simulink model "uvms_kinematics"  (Simulink 7.9)
settings: Solver=ode3  StartTime=0.0  StopTime=10.0  FixedStep=dt  RelTol=1e-3
values from neighbouring files (symbols this model uses):
  DH = struct('a',zeros(n,1),'d',zeros(n,1),'alpha',zeros(n,1))    [init.m]
  dt = 0.01    [run_simulation.m]
  VV_States = struct('StatusLinear',0, 'StatusAngular', 0 ,'Circle2EEVec',zeros(3,1), 'linearVehicleVelocity', zeros(6,1),                     'angularVehicleVelocity', zeros(6,1) , 'psibe',0, 'V_EE', zeros(6,1), 'VdotP',0)    [run_simulation.m]
undefined symbols (not defined in the file or in its folder): CircleProps, ee_pose_init, ee_pose_quaternion_init, q_init, QLimits, vehicle_euler_init, vehicle_position_init
libraries: simulink x6
settings Model: Creator=simena  LastModifiedBy=simena
settings DebuggingCC: UnderspecifiedInitializationDetection=Simplified

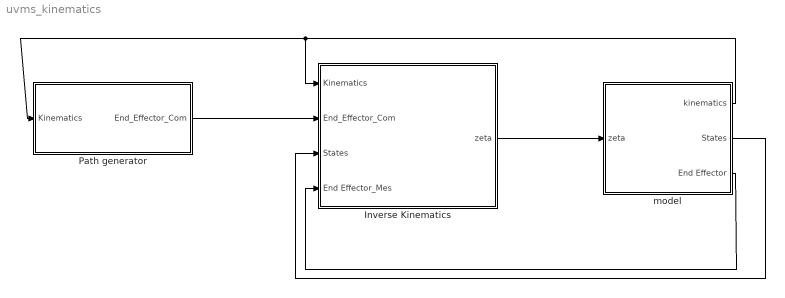
== system uvms_kinematics ==
  Inverse Kinematics : Subsystem
  Path generator : Subsystem
  model : Subsystem
  wires:
  Inverse Kinematics/1(zeta) -> model/1(zeta)
  model/1(kinematics) -> Inverse Kinematics/1(Kinematics), Path generator/1(Kinematics)
  model/3(End Effector) -> Inverse Kinematics/4(End Effector_Mes)
  Path generator/1(End_Effector_Com) -> Inverse Kinematics/2(End_Effector_Com)
  model/2(States) -> Inverse Kinematics/3(States)

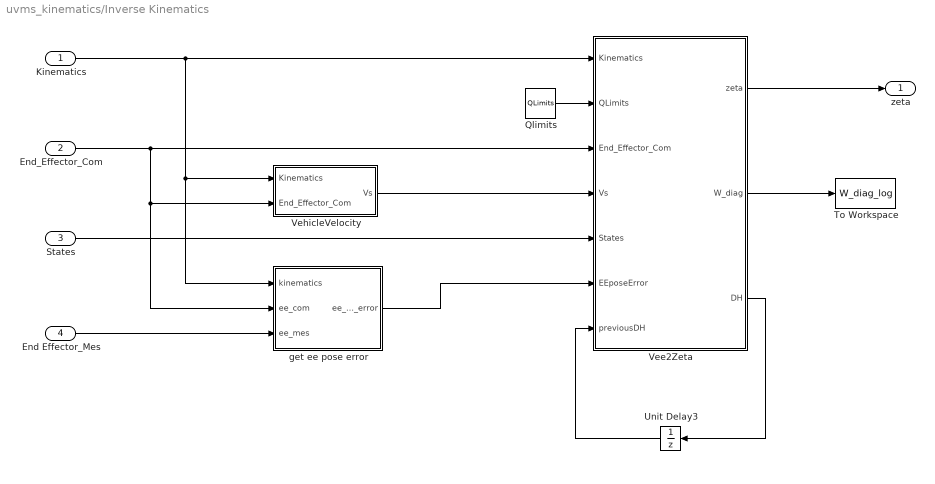
== system uvms_kinematics/Inverse Kinematics ==
  Kinematics : Inport
  End_Effector_Com : Inport  Port=2
  States : Inport  Port=3
  End Effector_Mes : Inport  Port=4
  Qlimits : Constant  Value=QLimits  OutDataTypeStr=Bus: qlimits_bus
  To Workspace : ToWorkspace  VariableName=W_diag_log  SampleTime=-1  SaveFormat=Timeseries
  Unit Delay3 : UnitDelay  X0=zeros(12,12)  SampleTime=-1
  Vee2Zeta : MATLAB Function  TreatAsAtomicUnit=on  SystemSampleTime=dt
  VehicleVelocity : Subsystem
  get ee pose error : Subsystem
  zeta : Outport
  wires:
  Qlimits/1 -> Vee2Zeta/2(QLimits)
  Unit Delay3/1 -> Vee2Zeta/7(previousDH)
  VehicleVelocity/1(Vs) -> Vee2Zeta/4(Vs)
  States/1 -> Vee2Zeta/5(States)
  End Effector_Mes/1 -> get ee pose error/3(ee_mes)
  Vee2Zeta/1(zeta) -> zeta/1
  get ee pose error/1(ee_pose_error) -> Vee2Zeta/6(EEposeError)
  Vee2Zeta/2(W_diag) -> To Workspace/1
  Vee2Zeta/3(DH) -> Unit Delay3/1
  Kinematics/1 -> Vee2Zeta/1(Kinematics), get ee pose error/1(kinematics), VehicleVelocity/1(Kinematics)
  End_Effector_Com/1 -> Vee2Zeta/3(End_Effector_Com), VehicleVelocity/2(End_Effector_Com), get ee pose error/2(ee_com)

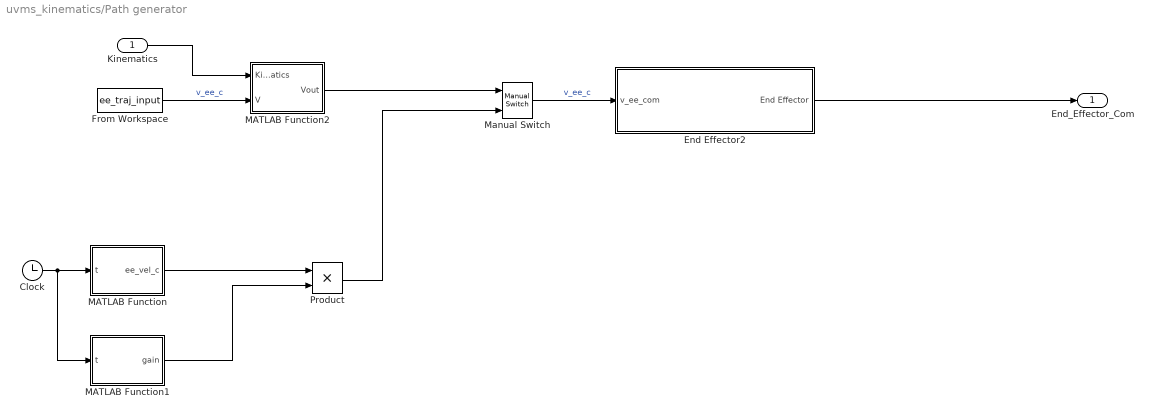
== system uvms_kinematics/Path generator ==
  Kinematics : Inport
  Clock : Clock
  End Effector2 : Subsystem
  From Workspace : FromWorkspace  VariableName=ee_traj_input  SampleTime=0
  MATLAB Function : MATLAB Function  TreatAsAtomicUnit=on
  MATLAB Function1 : MATLAB Function  TreatAsAtomicUnit=on
  MATLAB Function2 : MATLAB Function  TreatAsAtomicUnit=on
  Manual Switch : simulink/Signal Routing/Manual Switch  sw=1  action=0  varsize=off
  Product : Product  RndMeth=Zero
  End_Effector_Com : Outport
  wires:
  From Workspace/1 -> MATLAB Function2/2(V)  "v_ee_c"
  Clock/1 -> MATLAB Function/1(t), MATLAB Function1/1(t)
  MATLAB Function/1(ee_vel_c) -> Product/1
  Product/1 -> Manual Switch/2
  MATLAB Function1/1(gain) -> Product/2
  Manual Switch/1 -> End Effector2/1(v_ee_com)  "v_ee_c"
  End Effector2/1(End Effector) -> End_Effector_Com/1
  MATLAB Function2/1(Vout) -> Manual Switch/1
  Kinematics/1 -> MATLAB Function2/1(Kinematics)

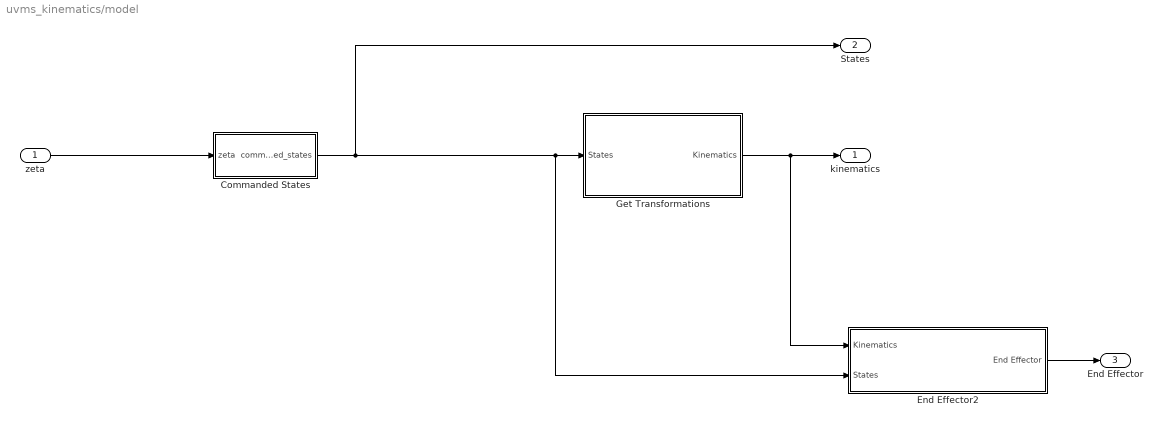
== system uvms_kinematics/model ==
  zeta : Inport
  Commanded States : Subsystem
  End Effector2 : Subsystem
  Get Transformations : Subsystem
  kinematics : Outport
  States : Outport  Port=2
  End Effector : Outport  Port=3
  wires:
  Get Transformations/1(Kinematics) -> End Effector2/1(Kinematics), kinematics/1
  Commanded States/1(commanded_states) -> Get Transformations/1(States), End Effector2/2(States), States/1
  zeta/1 -> Commanded States/1(zeta)
  End Effector2/1(End Effector) -> End Effector/1

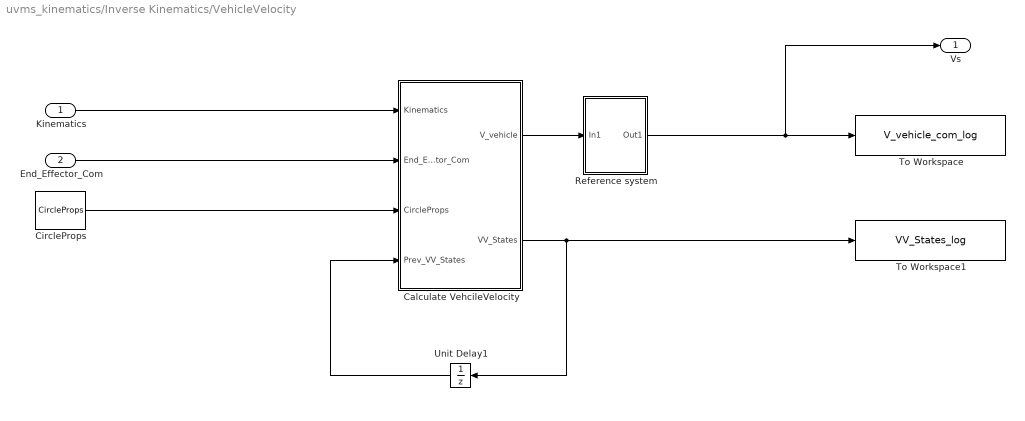
== system uvms_kinematics/Inverse Kinematics/VehicleVelocity ==
  Kinematics : Inport
  End_Effector_Com : Inport  Port=2
  Calculate VehcileVelocity : MATLAB Function  TreatAsAtomicUnit=on  SystemSampleTime=dt
  CircleProps : Constant  Value=CircleProps  OutDataTypeStr=Bus: circleProps_bus
  Reference system : Subsystem
  To Workspace : ToWorkspace  VariableName=V_vehicle_com_log  SampleTime=-1  SaveFormat=Timeseries
  To Workspace1 : ToWorkspace  VariableName=VV_States_log  SampleTime=-1  SaveFormat=Timeseries
  Unit Delay1 : UnitDelay  X0=VV_States  SampleTime=dt
  Vs : Outport
  wires:
  CircleProps/1 -> Calculate VehcileVelocity/3(CircleProps)
  Unit Delay1/1 -> Calculate VehcileVelocity/4(Prev_VV_States)
  Kinematics/1 -> Calculate VehcileVelocity/1(Kinematics)
  End_Effector_Com/1 -> Calculate VehcileVelocity/2(End_Effector_Com)
  Calculate VehcileVelocity/2(VV_States) -> Unit Delay1/1, To Workspace1/1
  Calculate VehcileVelocity/1(V_vehicle) -> Reference system/1(In1)
  Reference system/1(Out1) -> Vs/1, To Workspace/1

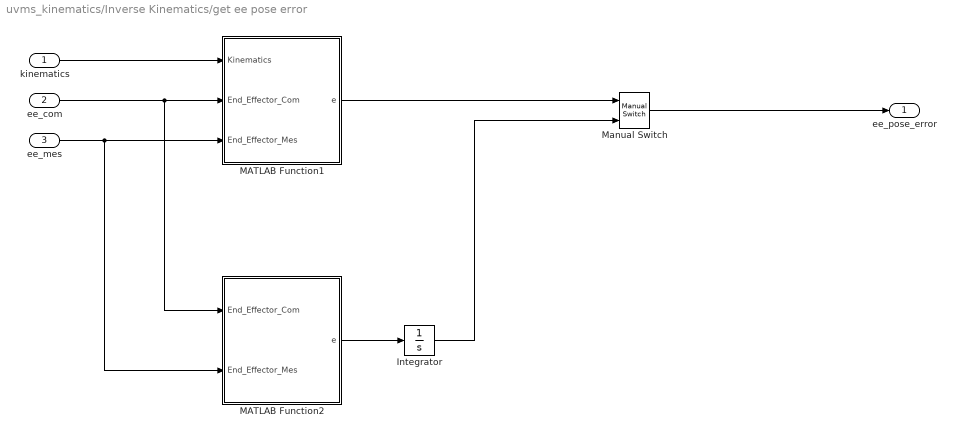
== system uvms_kinematics/Inverse Kinematics/get ee pose error ==
  kinematics : Inport
  ee_com : Inport  Port=2
  ee_mes : Inport  Port=3
  Integrator : Integrator
  MATLAB Function1 : MATLAB Function  TreatAsAtomicUnit=on
  MATLAB Function2 : MATLAB Function  TreatAsAtomicUnit=on
  Manual Switch : simulink/Signal Routing/Manual Switch  sw=0  action=0  varsize=off
  ee_pose_error : Outport
  wires:
  ee_com/1 -> MATLAB Function1/2(End_Effector_Com), MATLAB Function2/1(End_Effector_Com)
  ee_mes/1 -> MATLAB Function1/3(End_Effector_Mes), MATLAB Function2/2(End_Effector_Mes)
  kinematics/1 -> MATLAB Function1/1(Kinematics)
  MATLAB Function1/1(e) -> Manual Switch/1
  Manual Switch/1 -> ee_pose_error/1
  MATLAB Function2/1(e) -> Integrator/1
  Integrator/1 -> Manual Switch/2

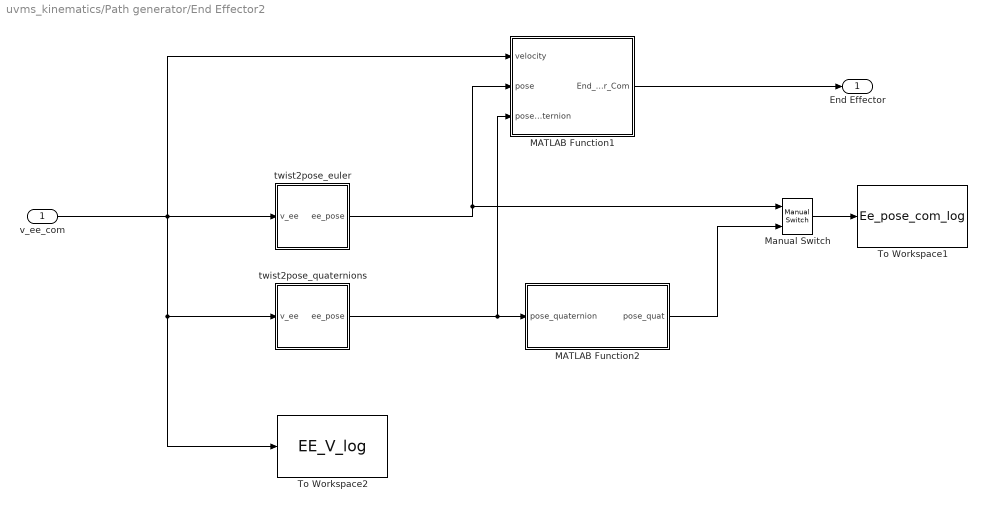
== system uvms_kinematics/Path generator/End Effector2 ==
  v_ee_com : Inport
  MATLAB Function1 : MATLAB Function  TreatAsAtomicUnit=on
  MATLAB Function2 : MATLAB Function  TreatAsAtomicUnit=on
  Manual Switch : simulink/Signal Routing/Manual Switch  sw=0  action=0  varsize=off
  To Workspace1 : ToWorkspace  VariableName=Ee_pose_com_log  SampleTime=dt  SaveFormat=Timeseries
  To Workspace2 : ToWorkspace  VariableName=EE_V_log  SampleTime=dt  SaveFormat=Timeseries
  twist2pose_euler : Subsystem
  twist2pose_quaternions : Subsystem
  End Effector : Outport
  wires:
  twist2pose_euler/1(ee_pose) -> MATLAB Function1/2(pose), Manual Switch/1
  MATLAB Function1/1(End_Effector_Com) -> End Effector/1
  twist2pose_quaternions/1(ee_pose) -> MATLAB Function1/3(pose_quaternion), MATLAB Function2/1(pose_quaternion)
  v_ee_com/1 -> twist2pose_euler/1(v_ee), MATLAB Function1/1(velocity), twist2pose_quaternions/1(v_ee), To Workspace2/1
  Manual Switch/1 -> To Workspace1/1
  MATLAB Function2/1(pose_quat) -> Manual Switch/2

== system uvms_kinematics/model/Commanded States ==
  zeta : Inport
  To Workspace : ToWorkspace  VariableName=commanded_states_log  SampleTime=-1  SaveFormat=Timeseries
  commanded states : Subsystem  TreatAsAtomicUnit=on
  commanded_states : Outport
  wires:
  zeta/1 -> commanded states/1(zeta)
  commanded states/1(commanded_states) -> commanded_states/1, To Workspace/1

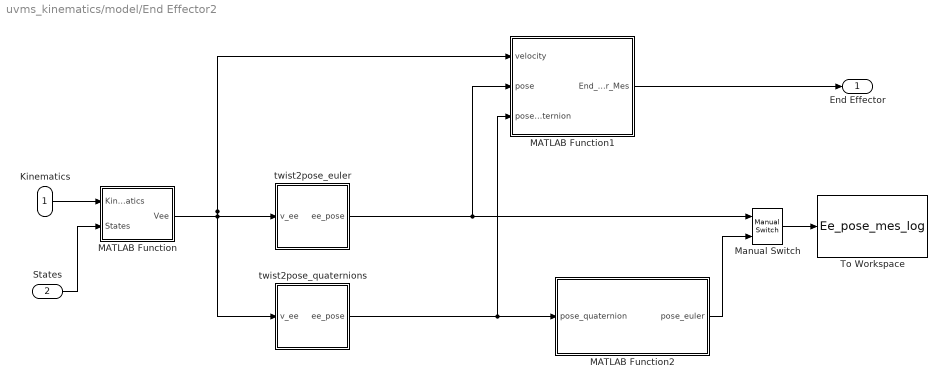
== system uvms_kinematics/model/End Effector2 ==
  Kinematics : Inport
  States : Inport  Port=2
  MATLAB Function : MATLAB Function  TreatAsAtomicUnit=on
  MATLAB Function1 : MATLAB Function  TreatAsAtomicUnit=on
  MATLAB Function2 : MATLAB Function  TreatAsAtomicUnit=on
  Manual Switch : simulink/Signal Routing/Manual Switch  sw=1  action=0  varsize=off
  To Workspace : ToWorkspace  VariableName=Ee_pose_mes_log  SampleTime=dt  SaveFormat=Timeseries
  twist2pose_euler : Subsystem
  twist2pose_quaternions : Subsystem
  End Effector : Outport
  wires:
  twist2pose_euler/1(ee_pose) -> MATLAB Function1/2(pose), Manual Switch/1
  Kinematics/1 -> MATLAB Function/1(Kinematics)
  States/1 -> MATLAB Function/2(States)
  MATLAB Function/1(Vee) -> twist2pose_euler/1(v_ee), MATLAB Function1/1(velocity), twist2pose_quaternions/1(v_ee)
  MATLAB Function1/1(End_Effector_Mes) -> End Effector/1
  twist2pose_quaternions/1(ee_pose) -> MATLAB Function1/3(pose_quaternion), MATLAB Function2/1(pose_quaternion)
  MATLAB Function2/1(pose_euler) -> Manual Switch/2
  Manual Switch/1 -> To Workspace/1

== system uvms_kinematics/model/Get Transformations ==
  States : Inport
  DH parameters : Constant  Value=DH  OutDataTypeStr=Bus: DH_bus
  Jacobians : MATLAB Function  TreatAsAtomicUnit=on  SystemSampleTime=dt
  Transformations : MATLAB Function  TreatAsAtomicUnit=on  SystemSampleTime=dt
  Kinematics : Outport
  wires:
  DH parameters/1 -> Transformations/2(DH)  "DH"
  Transformations/1(Ti) -> Jacobians/1(Ti)
  States/1 -> Transformations/1(States)
  Jacobians/1(Kinematics) -> Kinematics/1

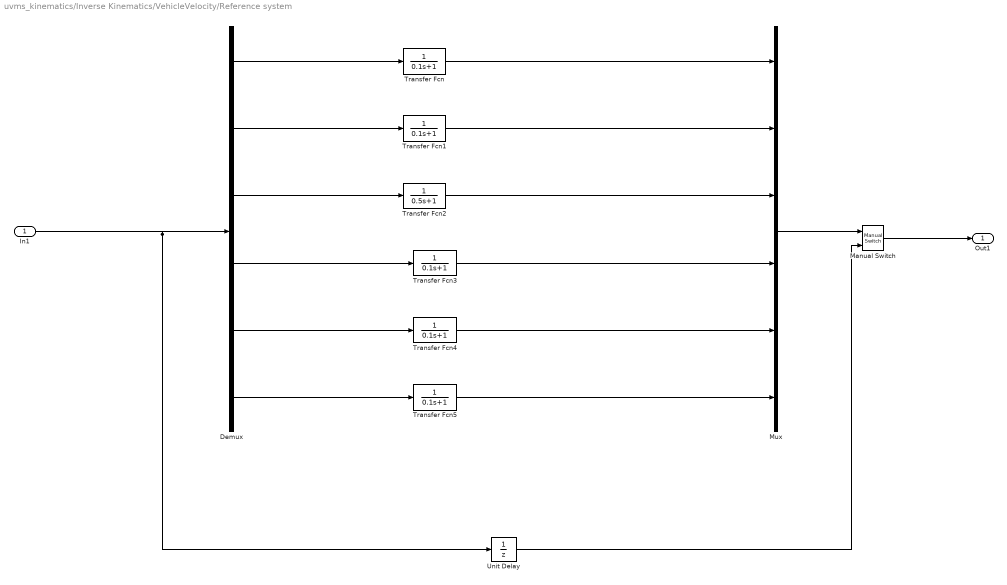
== system uvms_kinematics/Inverse Kinematics/VehicleVelocity/Reference system ==
  In1 : Inport
  Demux : Demux  Outputs=6
  Manual Switch : simulink/Signal Routing/Manual Switch  sw=0  action=0  varsize=off
  Mux : Mux  Inputs=6
  Transfer Fcn{,1,3..5} (5 alike) : TransferFcn  Denominator=[0.1 1]
  Transfer Fcn2 : TransferFcn  Denominator=[0.5 1]
  Unit Delay : UnitDelay  SampleTime=-1
  Out1 : Outport
  wires:
  Mux/1 -> Manual Switch/1
  Manual Switch/1 -> Out1/1
  In1/1 -> Demux/1, Unit Delay/1
  Unit Delay/1 -> Manual Switch/2
  Demux/1 -> Transfer Fcn/1
  Demux/2 -> Transfer Fcn1/1
  Demux/3 -> Transfer Fcn2/1
  Transfer Fcn/1 -> Mux/1
  Transfer Fcn1/1 -> Mux/2
  Transfer Fcn2/1 -> Mux/3
  Demux/4 -> Transfer Fcn3/1
  Demux/5 -> Transfer Fcn4/1
  Demux/6 -> Transfer Fcn5/1
  Transfer Fcn3/1 -> Mux/4
  Transfer Fcn4/1 -> Mux/5
  Transfer Fcn5/1 -> Mux/6

== system uvms_kinematics/Path generator/End Effector2/twist2pose_euler ==
  v_ee : Inport
  Demux : Demux  Outputs=2
  Integrator : Integrator  InitialCondition=ee_pose_init
  Mux : Mux  Inputs=2
  body2eulervel : MATLAB Function  TreatAsAtomicUnit=on  SystemSampleTime=dt
  ee_pose : Outport
  wires:
  v_ee/1 -> body2eulervel/1(ee_velocity_twist)
  body2eulervel/1(ee_rates) -> Integrator/1
  Integrator/1 -> Demux/1
  Demux/2 -> body2eulervel/2(euler_angles_ee), Mux/2  "ee_angle"
  Demux/1 -> Mux/1  "ee_pos"
  Mux/1 -> ee_pose/1

== system uvms_kinematics/Path generator/End Effector2/twist2pose_quaternions ==
  v_ee : Inport
  Integrator : Integrator  InitialCondition=ee_pose_quaternion_init
  MATLAB Function : MATLAB Function  TreatAsAtomicUnit=on
  body2quat : MATLAB Function  TreatAsAtomicUnit=on  SystemSampleTime=dt
  ee_pose : Outport
  wires:
  v_ee/1 -> body2quat/1(ee_velocity_twist)
  body2quat/1(ee_rates) -> Integrator/1
  Integrator/1 -> MATLAB Function/1(poseIn)
  MATLAB Function/1(pose) -> ee_pose/1
  MATLAB Function/2(quaternion) -> body2quat/2(quat)

== system uvms_kinematics/model/Commanded States/commanded states ==
  zeta : Inport
  Measure States : MATLAB Function  TreatAsAtomicUnit=on
  Reference system : Subsystem
  get dzeta : Subsystem
  zeta2xi : Subsystem
  commanded_states : Outport
  wires:
  Measure States/1(Commanded_States) -> commanded_states/1
  zeta2xi/1(xi) -> Measure States/3(xi)
  zeta/1 -> Reference system/1(zeta in)
  Reference system/1(zeta_out) -> Measure States/2(zeta), get dzeta/1(zeta), zeta2xi/1(zeta)
  get dzeta/1(dzeta) -> Measure States/1(dzeta)

== system uvms_kinematics/model/End Effector2/twist2pose_euler ==
  v_ee : Inport
  Demux : Demux  Outputs=2
  Integrator : Integrator  InitialCondition=ee_pose_init
  Mux : Mux  Inputs=2
  body2eulervel : MATLAB Function  TreatAsAtomicUnit=on  SystemSampleTime=dt
  ee_pose : Outport
  wires:
  v_ee/1 -> body2eulervel/1(ee_velocity_twist)
  body2eulervel/1(ee_rates) -> Integrator/1
  Integrator/1 -> Demux/1
  Demux/2 -> body2eulervel/2(euler_angles_ee), Mux/2  "ee_angle"
  Demux/1 -> Mux/1  "ee_pos"
  Mux/1 -> ee_pose/1

== system uvms_kinematics/model/End Effector2/twist2pose_quaternions ==
  v_ee : Inport
  Integrator : Integrator  InitialCondition=ee_pose_quaternion_init
  MATLAB Function : MATLAB Function  TreatAsAtomicUnit=on
  body2quat : MATLAB Function  TreatAsAtomicUnit=on  SystemSampleTime=dt
  ee_pose : Outport
  wires:
  v_ee/1 -> body2quat/1(ee_velocity_twist)
  body2quat/1(ee_rates) -> Integrator/1
  Integrator/1 -> MATLAB Function/1(poseIn)
  MATLAB Function/1(pose) -> ee_pose/1
  MATLAB Function/2(quaternion) -> body2quat/2(quat)

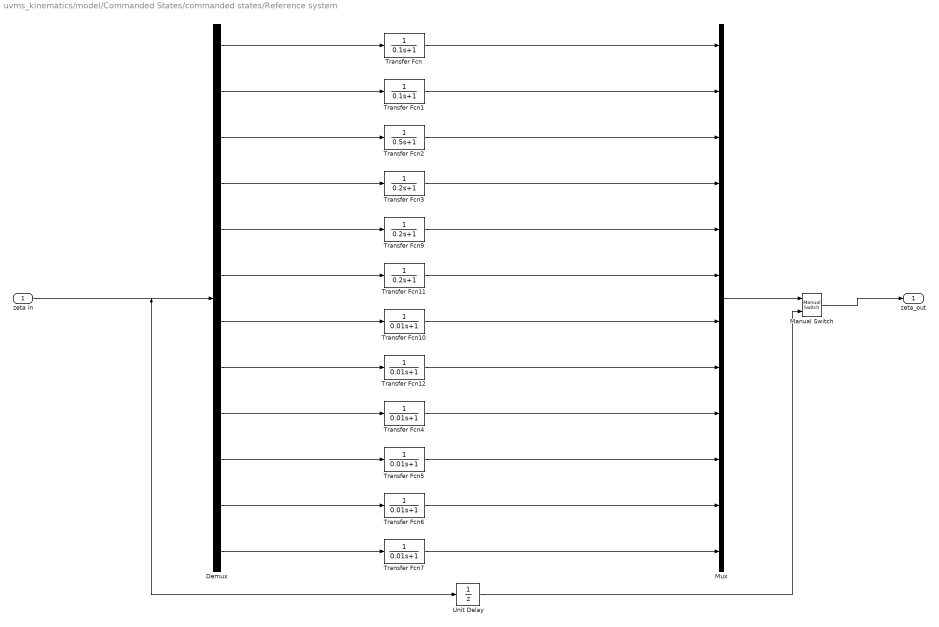
== system uvms_kinematics/model/Commanded States/commanded states/Reference system ==
  zeta in : Inport
  Demux : Demux  Outputs=12
  Manual Switch : simulink/Signal Routing/Manual Switch  sw=0  action=0  varsize=off
  Mux : Mux  Inputs=12
  Transfer Fcn : TransferFcn  Denominator=[0.1 1]
  Transfer Fcn1 : TransferFcn  Denominator=[0.1 1]
  Transfer Fcn{4..7,10,12} (6 alike) : TransferFcn  Denominator=[0.01 1]
  Transfer Fcn11 : TransferFcn  Denominator=[0.2 1]
  Transfer Fcn2 : TransferFcn  Denominator=[0.5 1]
  Transfer Fcn3 : TransferFcn  Denominator=[0.2 1]
  Transfer Fcn9 : TransferFcn  Denominator=[0.2 1]
  Unit Delay : UnitDelay  SampleTime=-1
  zeta_out : Outport
  wires:
  Demux/1 -> Transfer Fcn/1
  Transfer Fcn/1 -> Mux/1
  Demux/2 -> Transfer Fcn1/1
  Demux/3 -> Transfer Fcn2/1
  Demux/4 -> Transfer Fcn3/1
  Demux/5 -> Transfer Fcn9/1
  Demux/6 -> Transfer Fcn11/1
  Demux/7 -> Transfer Fcn10/1
  Demux/8 -> Transfer Fcn12/1
  Demux/9 -> Transfer Fcn4/1
  Demux/10 -> Transfer Fcn5/1
  Demux/11 -> Transfer Fcn6/1
  Demux/12 -> Transfer Fcn7/1
  Transfer Fcn1/1 -> Mux/2
  Transfer Fcn2/1 -> Mux/3
  Transfer Fcn3/1 -> Mux/4
  Transfer Fcn9/1 -> Mux/5
  Transfer Fcn11/1 -> Mux/6
  Transfer Fcn10/1 -> Mux/7
  Transfer Fcn12/1 -> Mux/8
  Transfer Fcn4/1 -> Mux/9
  Transfer Fcn5/1 -> Mux/10
  Transfer Fcn6/1 -> Mux/11
  Transfer Fcn7/1 -> Mux/12
  Mux/1 -> Manual Switch/1
  Manual Switch/1 -> zeta_out/1
  zeta in/1 -> Demux/1, Unit Delay/1
  Unit Delay/1 -> Manual Switch/2

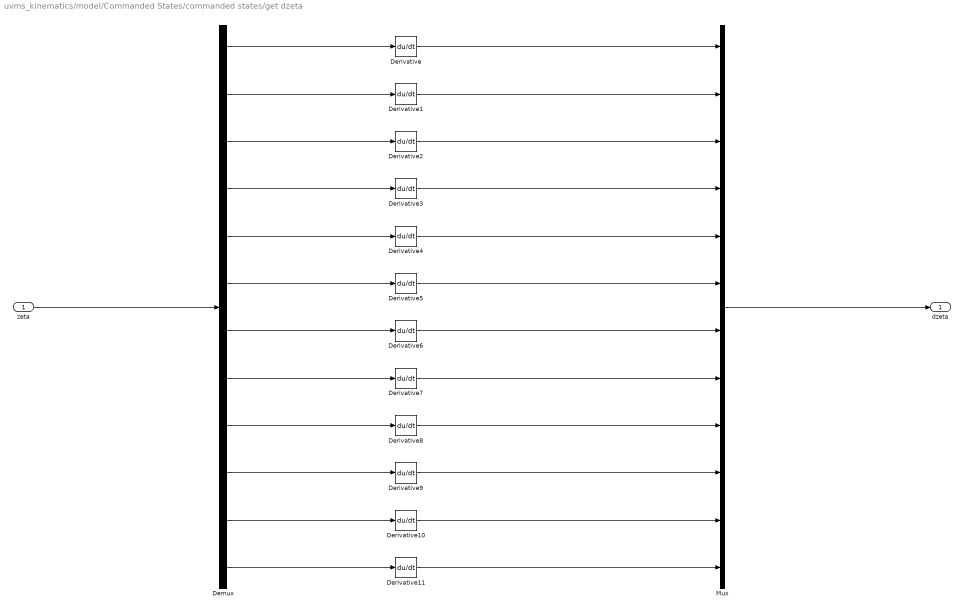
== system uvms_kinematics/model/Commanded States/commanded states/get dzeta ==
  zeta : Inport
  Demux : Demux  Outputs=12
  Derivative{,1..11} (12 alike) : Derivative
  Mux : Mux  Inputs=12
  dzeta : Outport
  wires:
  Demux/1 -> Derivative/1
  zeta/1 -> Demux/1
  Derivative/1 -> Mux/1
  Demux/2 -> Derivative1/1
  Demux/3 -> Derivative2/1
  Demux/4 -> Derivative3/1
  Demux/5 -> Derivative4/1
  Demux/6 -> Derivative5/1
  Demux/7 -> Derivative6/1
  Demux/8 -> Derivative7/1
  Demux/9 -> Derivative8/1
  Demux/10 -> Derivative9/1
  Demux/11 -> Derivative10/1
  Demux/12 -> Derivative11/1
  Derivative1/1 -> Mux/2
  Derivative2/1 -> Mux/3
  Derivative3/1 -> Mux/4
  Derivative4/1 -> Mux/5
  Derivative5/1 -> Mux/6
  Derivative6/1 -> Mux/7
  Derivative7/1 -> Mux/8
  Derivative8/1 -> Mux/9
  Derivative9/1 -> Mux/10
  Derivative10/1 -> Mux/11
  Derivative11/1 -> Mux/12
  Mux/1 -> dzeta/1

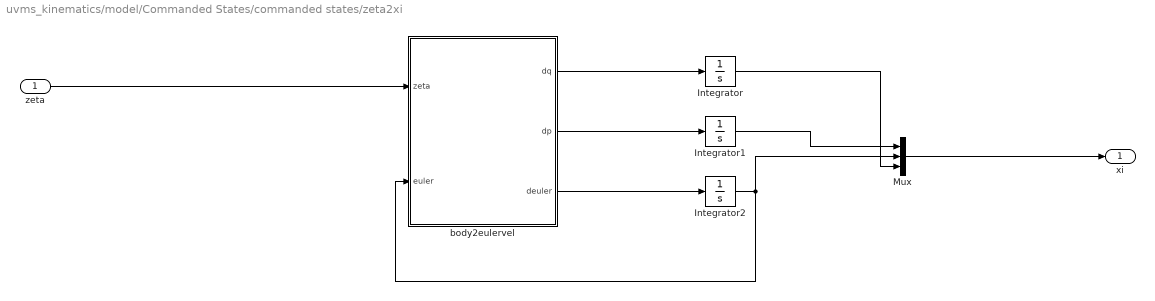
== system uvms_kinematics/model/Commanded States/commanded states/zeta2xi ==
  zeta : Inport
  Integrator : Integrator  InitialCondition=q_init
  Integrator1 : Integrator  InitialCondition=vehicle_position_init
  Integrator2 : Integrator  InitialCondition=vehicle_euler_init
  Mux : Mux  Inputs=3
  body2eulervel : MATLAB Function  TreatAsAtomicUnit=on  SystemSampleTime=dt
  xi : Outport
  wires:
  body2eulervel/1(dq) -> Integrator/1
  body2eulervel/2(dp) -> Integrator1/1
  body2eulervel/3(deuler) -> Integrator2/1
  zeta/1 -> body2eulervel/1(zeta)
  Integrator2/1 -> body2eulervel/2(euler), Mux/2
  Mux/1 -> xi/1
  Integrator1/1 -> Mux/1
  Integrator/1 -> Mux/3

== matlab function model/Get Transformations/Jacobians ==
  data: Ti input Bus: Ti_bus; Kinematics output Bus: kin_bus
function Kinematics  = getJacobians(Ti)
%#codegen
    n=6;
    Ji = struct('Ji',zeros(n,n+6,n),'Je',zeros(n,n+6),'Jbe',zeros(n,n));
    Kinematics = struct('Ti', Ti, 'Ji',Ji);
    ji=zeros(6,6);
    for i=1:n
        ji=getji(Ti,i);
    
        Ji.Ji(:,:,i) = [Ti.Adgbi_inv(:,:,i), Ti.Adgbi_inv(:,:,i)*ji];
    end
    j6 = getje(Ti);
    Ji.Je = [Ti.Adgbe_inv, Ti.Adgbe_inv*j6];
    Ji.Jbe = Ti.Adgbe_inv*j6;
    Kinematics.Ji = Ji;
    Kinematics.Ti = Ti;
end




% return matrix Ji (see report)
function mat = getji(Ti,i)
    n=6;
    mat=zeros(6,6);
    Xii=[0,0,0,0,0,1]';
    mat(:,1)=eye(6)*Xii;
    for j=2:n
        if j<=i
            mat(:,j) = Ti.Adgbi(:,:,j-1)*Xii;
        end
    end

end

% return matrix Je (see report)
function mat = getje(Ti)
    n=6;
    mat=zeros(6,6);
    Xii=[0,0,0,0,0,1]';
    mat(:,1)=eye(6)*Xii;
    for i=2:(n-1)
        mat(:,i) = Ti.Adgbi(:,:,i-1)*Xii;
    end
    mat(:,6) = Ti.Adgbe*Xii;

end

function S = skew(v)
  S = [  0   -v(3)  v(2)
       v(3)  0    -v(1)
       -v(2) v(1)   0];
end

== matlab function model/Get Transformations/Transformations ==
  data: States input double; DH input Bus: DH_bus; Ti output Bus: Ti_bus
function Ti    = getTransformations(States,DH)
%#codegen
% Return transformations, rotations, positions and adjoint matrices for
% robot links
% Tbi.gbi(:,:,i) is the transformation from b to i etc
    n=6;    % number of links
    Xi = States.xi;
    q = Xi(7:12);
    eta = Xi(1:6);
           
    Ti = struct('g0b',zeros(4,4),'g0i',zeros(4,4,n),'R0i', zeros(3,3,n),'R0b',zeros(3,3),'p0i', zeros(3,1,n), 'Adg0i',zeros(6,6,n),'Adg0i_inv',zeros(6,6,n),   ...
    'gbi',zeros(4,4,n),'Rbi', zeros(3,3,n),'pbi', zeros(3,1,n),'Adgbi',zeros(6,6,n),'Adgbi_inv',zeros(6,6,n),...
    'g6e',eye(4) ,'g0e',zeros(4,4),'R0e', zeros(3,3),'p0e', zeros(3,1),  'Adg0e',zeros(6,6),'Adg0e_inv',zeros(6,6),   ...
    'gbe',zeros(4,4),'Rbe', zeros(3,3),'pbe', zeros(3,1),'Adgbe',zeros(6,6),'Adgbe_inv',zeros(6,6) ...
    );
      
    Ti.g6e = DH.g6e;
    Ti.g0b=eta2g0b(eta);
    
    
    Ti.R0b = Ti.g0b(1:3,1:3);

    % initial matrices 
    g=eye(4);
    g0=Ti.g0b;
    
    for i=1:n
       % transformations from frame b to frame i
       Ti.gbi(:,:,i) = g*getHom(q,DH,i);
       Ti.Rbi(:,:,i) = getRot(Ti.gbi(:,:,i));
       Ti.pbi(:,:,i) = getPos(Ti.gbi(:,:,i));
       Ti.Adgbi(:,:,i) = getAdgbi(Ti.Rbi(:,:,i), Ti.pbi(:,:,i) );
       Ti.Adgbi_inv(:,:,i) = getAdgbi_inv(Ti.Rbi(:,:,i), Ti.pbi(:,:,i) );
       g=Ti.gbi(:,:,i);
       % transformations from frame 0 to frame i
       Ti.g0i(:,:,i) = g0*getHom(q,DH,i);
       Ti.R0i(:,:,i) = getRot(Ti.g0i(:,:,i));
       Ti.p0i(:,:,i) = getPos(Ti.g0i(:,:,i));
       Ti.Adg0i(:,:,i) = getAdgbi(Ti.R0i(:,:,i), Ti.p0i(:,:,i) );
       Ti.Adg0i_inv(:,:,i) = getAdgbi_inv(Ti.R0i(:,:,i), Ti.p0i(:,:,i) );
       g0=Ti.g0i(:,:,i);
    end
    
    % transformation from frame 0 to ee
    g0e = Ti.g0i(:,:,6)*Ti.g6e;
    Ti.g0e = g0e;
    Ti.R0e = getRot(g0e);
    Ti.p0e = getPos(g0e);
    Ti.Adg0e = getAdgbi(Ti.R0e, Ti.p0e );
    Ti.Adg0e_inv = getAdgbi_inv(Ti.R0e, Ti.p0e);
        
    % transformation from frame b to ee
    gbe = Ti.gbi(:,:,6)*Ti.g6e;
    Ti.gbe = gbe;
    Ti.Rbe = getRot(gbe);
    Ti.pbe = getPos(gbe);
    Ti.Adgbe = getAdgbi(Ti.Rbe , Ti.pbe );
    Ti.Adgbe_inv = getAdgbi_inv(Ti.Rbe , Ti.pbe );
    
    % DEBUG
    % coder.extrinsic('disp');
    % coder.extrinsic('num2str');
    %if counter == 12        
%         disp(['------iteration: ' num2str(counter)]);
%         q';
%         [phi, theta,psi]=myR2euler(Ti.R0i(:,:,1))
%         Ti.g0i(:,:,1)
       %Ti.Adgbi(:,:,1)
       %Ti.Adgbi_inv(:,:,1)
       %Ti.pbi(:,1)
       %Ti.p0i(:,1)
       
    %end
    
 end




% homogenous transformation matrix - DH convention
% mat=Rot_z(theta)Trans_z(d)Trans_x(a)Rot_x(alpha)
function mat=getHom(q,DH,i)
    alpha=DH.alpha(i);
    a=DH.a(i);
    d=DH.d(i);
    theta=q(i);
    mat=eye(4);
    mat=[cos(theta), -sin(theta)*cos(alpha), sin(theta)*sin(alpha), a*cos(theta);
         sin(theta), cos(theta)*cos(alpha), -cos(theta)*sin(alpha), a*sin(theta);
         0, sin(alpha), cos(alpha), d;
         0,0,0,1
    ];

end

% extract position from homogenous 
% matrix
function vec = getPos(g)
    vec=g(1:3,4);
end

% extract rotation matrix-part out of
% homogenous matrix
function mat = getRot(g)
    mat=g(1:3,1:3);
end

function mat = getAdgbi(R,p)
    mat = zeros(6,6);
    ps=skew(p);
    mat=[R , ps*R ; zeros(3,3), R ];
end

function mat = getAdgbi_inv(R,p)
    mat = zeros(6,6);
    Rt=transpose(R);
    ps=skew(p);
    mat=[Rt , -Rt*ps ; zeros(3,3), Rt ];
end

function [phi,theta,psi] = myR2euler(R)
    phi   = atan2(R(3,2),R(3,3));
    theta = -asin(R(3,1));
    psi   = atan2(R(2,1),R(1,1));
end

function mat = eta2g0b(eta)
    mat = zeros(4,4);
    R=Rzyx(eta(4),eta(5),eta(6));
    pos=[eta(1); eta(2); eta(3)];
    mat = [R,pos;0,0,0,1];
end

function R = Rzyx(phi,theta,psi)
    cphi = cos(phi);
    sphi = sin(phi);
    cth  = cos(theta);
    sth  = sin(theta);
    cpsi = cos(psi);
    spsi = sin(psi);
    R = [...
       cpsi*cth  -spsi*cphi+cpsi*sth*sphi  spsi*sphi+cpsi*cphi*sth
       spsi*cth  cpsi*cphi+sphi*sth*spsi   -cpsi*sphi+sth*spsi*cphi
       -sth      cth*sphi                  cth*cphi ];
end



function S = skew(v)
  S = [  0   -v(3)  v(2)
       v(3)  0    -v(1)
       -v(2) v(1)   0];
end

== matlab function model/End Effector2/twist2pose_euler/body2eulervel ==
  data: ee_velocity_twist input double size=6; ee_rates output double size=6; euler_angles_ee input double size=3
function ee_rates = fcn(ee_velocity_twist, euler_angles_ee)                       
    %#codegen
       
    phi=euler_angles_ee(1);
    theta=euler_angles_ee(2);
    psi=euler_angles_ee(3);
    
    
    cphi = cos(phi);
    sphi = sin(phi);
    cth  = cos(theta);
    sth  = sin(theta);
 
    J1 = Rzyx(phi,theta,psi);
 
    if cth==0, error('J2 is singular for theta = +-90 degrees'); end
 
    J2 = [...
      1  sphi*sth/cth  cphi*sth/cth;
      0  cphi          -sphi;
      0  sphi/cth      cphi/cth ];
 
    J = [ J1  zeros(3,3);
      zeros(3,3) J2 ];
        
    ee_rates = zeros(6,1);
    ee_rates=J*ee_velocity_twist;
end



function R = Rzyx(phi,theta,psi)
    cphi = cos(phi);
    sphi = sin(phi);
    cth  = cos(theta);
    sth  = sin(theta);
    cpsi = cos(psi);
    spsi = sin(psi);

    R = [...
       cpsi*cth  -spsi*cphi+cpsi*sth*sphi  spsi*sphi+cpsi*cphi*sth
       spsi*cth  cpsi*cphi+sphi*sth*spsi   -cpsi*sphi+sth*spsi*cphi
       -sth      cth*sphi                  cth*cphi ];
end

== matlab function Inverse Kinematics/Vee2Zeta ==
  data: Kinematics input double; QLimits input Bus: qlimits_bus; zeta output double; W_diag output double; End_Effector_Com input double; Vs input double; States input double; EEposeError input double size=6; previousDH input double; DH output double
function [zeta,W_diag,DH] = getZeta(Kinematics,QLimits,End_Effector_Com,Vs,  States,  EEposeError, previousDH)
%
%  Vp is the primary task trajectory - end effector
%  Vs is the secondary task trajectory - vehicle
%
%#codegen
    Jp = Kinematics.Ji.Je;
    Js = [eye(6), zeros(6,6)];
    xi = States.xi;
    q = xi (7:12);
    Ks = diag([   ones(1,3)*10  ,  ones(1,3)*80]);
    Vp = End_Effector_Com.velocity;
    
    [W, DH] = getW(q,previousDH,QLimits);
    
    %coder.extrinsic('disp');
    %disp('W is disabled in getZeta');
    %W = diag([ones(6,1)*100000 ; ones(6,1)]);
    
    JpInv = zeros(12,6);
    JsInv = zeros(12,6);
    %JsInv = pinv(Js);
    JsInv(:,:) = W \ transpose(Js) /((Js /W) *transpose(Js));
    JpInv(:,:) = W \ transpose(Jp) /((Jp /W) *transpose(Jp));
    I = eye(12);
    zeta = JpInv*(Vp + Ks*EEposeError  ) + ( I - JpInv*Jp) * JsInv * Vs;
    W_diag = diag(W);
end

% --------------------------------------------------------------------------
%   Returns the weighting matrix for use in the weighted pseudo inverse
% --------------------------------------------------------------------------
function [W, DH] = getW(q, previousDH,QLimits)
%#codegen    
% link joints
    DH =diag([ones(1,6)*2000,zeros(1,6)]); % derivative of H matrix
    qmin = QLimits.qmin;
    qmax = QLimits.qmax;
    for i=1:6
        temp = abs((((qmax(i)-qmin(i)).^2)*(2*q(i)-qmax(i)-qmin(i))) ./ ((4*(qmax(i)-q(i)).^2) * ((q(i)-qmin(i)).^2)));
        if (temp-previousDH(i+6,i+6)) < 0 
            DH(i+6,i+6)=abs(temp); % 0;
        else
            DH(i+6,i+6)=abs(temp);
        end
    end
   W = eye(12);
   W = W + DH;
   
end

== matlab function Path generator/MATLAB Function ==
  data: t input double; ee_vel_c output double
function ee_vel_c = fcn(t)
%#codegen
ee_vel_c = zeros(6,1);
% xvel = 0.2*cos(t/20);
% zvel = 0.2*sin(t);
% yvel = 0.3*cos(t/0.5);
% ee_vel_c(6) = 0.01*sin(t/30);
% ee_vel_c(1) = xvel;
% ee_vel_c(2) = yvel;
% ee_vel_c(3) = zvel;

ee_vel_c(3) = -0.1*sin(t);
ee_vel_c(5) = 0.7*sin(t);
ee_vel_c(6) = 0.7*sin(t);
ee_vel_c(4) = 0.7*sin(t);

%ee_vel_c(2) = 0.19;


%ee_vel_c(5) = 0.7*sin(t);

end

== matlab function Path generator/End Effector2/MATLAB Function2 ==
  data: pose_quat output double; pose_quaternion input double
function pose_quat = q2euler(pose_quaternion)
%#codegen
% [phi,theta,psi] = Q2EULER(q) computes the Euler angles from the unit 
% quaternions q = [eta eps1 eps2 eps3]
%
% Author:   Thor I. Fossen
% Date:      2001-06-14  
% Revisions: 2007-09-03  Test for singular solution theta = +-90 deg has been improved
% ________________________________________________________________
%
% MSS GNC is a Matlab toolbox for guidance, navigation and control.
% The toolbox is part of the Marine Systems Simulator (MSS).
%
% Copyright (C) 2008 Thor I. Fossen and Tristan Perez
% 
% This program is free software: you can redistribute it and/or modify
% it under the terms of the GNU General Public License as published by
% the Free Software Foundation, either version 3 of the License, or
% (at your option) any later version.
% 
% This program is distributed in the hope that it will be useful, but
% WITHOUT ANY WARRANTY; without even the implied warranty of
% MERCHANTABILITY or FITNESS FOR A PARTICULAR PURPOSE.  See the 
% GNU General Public License for more details.
% 
% You should have received a copy of the GNU General Public License
% along with this program.  If not, see <http://www.gnu.org/licenses/>.
% 
% E-mail: contact@marinecontrol.org
% URL:    <http://www.marinecontrol.org>



q = pose_quaternion(4:7);

R = Rquat(q);
 
phi   = atan2(R(3,2),R(3,3));
theta = -asin(R(3,1));
psi   = atan2(R(2,1),R(1,1));

pose_quat = [pose_quaternion(1:3); phi; theta; psi];
end





function R = Rquat(q)
%#codegen
eta = q(1);
eps = q(2:4);
S = skew(eps);
R = eye(3) + 2*eta*S + 2*S^2;

end

== matlab function model/End Effector2/MATLAB Function ==
  data: Kinematics input double; Vee output double; States input double
function Vee = fcn(Kinematics, States)
%#codegen
    Je = Kinematics.Ji.Je;    
    zeta = States.zeta;
    Vee = Je*zeta;
end

== matlab function model/End Effector2/MATLAB Function2 ==
  data: pose_euler output double; pose_quaternion input double
function pose_euler = q2euler(pose_quaternion)
%#codegen
% [phi,theta,psi] = Q2EULER(q) computes the Euler angles from the unit 
% quaternions q = [eta eps1 eps2 eps3]
%
% Author:   Thor I. Fossen
% Date:      2001-06-14  
% Revisions: 2007-09-03  Test for singular solution theta = +-90 deg has been improved
% ________________________________________________________________
%
% MSS GNC is a Matlab toolbox for guidance, navigation and control.
% The toolbox is part of the Marine Systems Simulator (MSS).
%
% Copyright (C) 2008 Thor I. Fossen and Tristan Perez
% 
% This program is free software: you can redistribute it and/or modify
% it under the terms of the GNU General Public License as published by
% the Free Software Foundation, either version 3 of the License, or
% (at your option) any later version.
% 
% This program is distributed in the hope that it will be useful, but
% WITHOUT ANY WARRANTY; without even the implied warranty of
% MERCHANTABILITY or FITNESS FOR A PARTICULAR PURPOSE.  See the 
% GNU General Public License for more details.
% 
% You should have received a copy of the GNU General Public License
% along with this program.  If not, see <http://www.gnu.org/licenses/>.
% 
% E-mail: contact@marinecontrol.org
% URL:    <http://www.marinecontrol.org>



q = pose_quaternion(4:7);

R = Rquat(q);
 
phi   = atan2(R(3,2),R(3,3));

if abs(R(3,1))>1.0 % error('solution is singular for theta = +- 90 degrees');
    R(3,1) = 0.99*sign(R(3,1))
end
theta = -asin(R(3,1));

psi   = atan2(R(2,1),R(1,1));

pose_euler = [pose_quaternion(1:3); phi; theta;psi];
end





function R = Rquat(q)
%#codegen
eta = q(1);
eps = q(2:4);
S = skew(eps);
R = eye(3) + 2*eta*S + 2*S^2;

end

== matlab function Inverse Kinematics/VehicleVelocity/Calculate VehcileVelocity ==
  data: Kinematics input double; End_Effector_Com input double; CircleProps input double; V_vehicle output double; Prev_VV_States input Bus: vehicleVelocityStates_bus; VV_States output Bus: vehicleVelocityStates_bus
function [V_vehicle , VV_States] = getVehicleVelocity(Kinematics,End_Effector_Com, CircleProps, Prev_VV_States)
%#codegen 
    %% set initial parameters
    VV_States = struct('StatusLinear',0, 'StatusAngular', 0 ,'Circle2EEVec',zeros(3,1), ...
                'linearVehicleVelocity', zeros(6,1), 'angularVehicleVelocity', zeros(6,1) , 'psibe',0, 'V_EE', zeros(6,1), 'VdotP', 0);
    V_vehicle = zeros(6,1);
    VV_States.V_EE = End_Effector_Com.velocity;
    VV_States.Circle2EEVec = getPCircle(Kinematics,CircleProps);    % vector from center of circle to EE
    VV_States.VdotP = ( Kinematics.Ti.Rbe * VV_States.V_EE(1:3) )' * VV_States.Circle2EEVec;
    VV_States.psibe = getPsibe( Kinematics);
    
    %% Get the status of the vehicle velocity assigner
    StatusLinear = getStatusLinear(Prev_VV_States,VV_States,CircleProps);
    StatusAngular = getStatusAngular(Prev_VV_States, VV_States, CircleProps); 
    
    %% act on the different StatusLinear
    if StatusLinear == 0 
        V_vehicle = zeros(6,1);
    elseif StatusLinear == 1
        V_vehicle = getLinearVelocitySameAsEE( VV_States, CircleProps, Kinematics);         
    elseif StatusLinear == 2
        V_vehicle = zeros(6,1);
    elseif StatusLinear == 3
        V_vehicle = getReturnToInnerCircleVelocity(VV_States,CircleProps, Kinematics);
    else
        error('something went wrong in linear states');
    end
    linearVelocity = V_vehicle;
    
    %% act on the different StatusAngular
    if StatusAngular == 0
        V_vehicle = zeros(6,1);
    elseif StatusAngular == 1 
        V_vehicle = getReturnToInnerpsibe(Kinematics, VV_States);
    else
        error('something went wrong in angular states');
    end
    angularVelocity = V_vehicle;
    
    %% set the statuses and the commanded vehicle
    V_vehicle = angularVelocity + linearVelocity;        
    VV_States.StatusLinear = StatusLinear;
    VV_States.StatusAngular = StatusAngular;
    VV_States.linearVehicleVelocity = linearVelocity;
    VV_States.angularVehicleVelocity = angularVelocity;       
end

%------------------------------------------------------------------------------------------------------------------
function V_vehicle = getReturnToInnerpsibe(Kinematics, VV_States)
    psibe = VV_States.psibe;
    k_ang = 1;
    Vee = VV_States.V_EE;
    omegabe = Vee(4:6);
    Rbe = Kinematics.Ti.Rbe;
    ybe = Kinematics.Ti.pbe(2);
    xbe = Kinematics.Ti.pbe(1);
    % angular velocity of ee around z axis vehicle
    rb0e = [0,0,1] * Rbe * omegabe;
    V_vehicle = [ybe ; -xbe ; 0 ; 0 ; 0 ; 1] * ( rb0e + k_ang * psibe  ) ;    
   
end

%------------------------------------------------------------------------------------------------------------------
function V_vehicle = getLinearVelocitySameAsEE(VV_States, CircleProps,Kinematics)
    Vee = VV_States.V_EE;
    Rbe = Kinematics.Ti.Rbe;
    x = norm(VV_States.Circle2EEVec )  - CircleProps.middleCircleRadius;
    radiusDelta = CircleProps.innerMiddelRadiusDelta;
    V_vehicle = zeros(6,1);
    V_vehicle(1:3) = Rbe*Vee(1:3)*(x/radiusDelta);
end

%------------------------------------------------------------------------------------------------------------------
function V_vehicle = getAngularSameAsEE(VV_States, Kinematics)
    Vee = VV_States.V_EE;
    omegabe = Vee(4:6);
    Rbe = Kinematics.Ti.Rbe;
    ybe = Kinematics.Ti.pbe(2);
    xbe = Kinematics.Ti.pbe(1);
    % angular velocity of ee around z axis vehicle
    rb0e = [0,0,1] * Rbe * omegabe;
    V_vehicle = [ybe ; -xbe ; 0 ; 0 ; 0 ; 1] * rb0e ;    
end

%------------------------------------------------------------------------------------------------------------------
% get the yaw angle by transforming the forward direction of the end
% effector (z) to the frame of the vehicle, and take the dot product
function psibe  = getPsibe( Kinematics)
    Rbe = Kinematics.Ti.Rbe;
    re = [0,0,1]';
    rb = Rbe * re;
    rb2 = rb(1:2);
    psibe = atan2 ( rb2(2) , rb2(1) );
end



%------------------------------------------------------------------------------------------------------------------
%   create a smooth velocity for the vehicle to make EE return to the inner
%   circle. 
function V_vehicle = getReturnToInnerCircleVelocity(VV_States , CircleProps, Kinematics)
    Vee = VV_States.V_EE;
    ir = CircleProps.innerCircleRadius;
    mr = CircleProps.middleCircleRadius;
    ve = Vee(1:3);
    Rbe = Kinematics.Ti.Rbe;
    c = ir + (mr - ir)./2;      % point between the two radiuses
    K = 0.6;
    V_vehicle = zeros(6,1);
    V_vehicle(1:3) = Rbe*ve +  K*VV_States.Circle2EEVec./norm( VV_States.Circle2EEVec );

end


%------------------------------------------------------------------------------------------------------------------
%  get the angular status 
%
function StatusAngular = getStatusAngular(Prev_VV_States, VV_States, CircleProps)
    PrevStatus = Prev_VV_States.StatusAngular;
    psibe = VV_States.psibe;
    prev_psibe = Prev_VV_States.psibe;
    
    if  PrevStatus == 0 && abs(psibe) >= CircleProps.psis
        StatusAngular = 1;
    elseif abs( psibe ) < CircleProps.psii
        StatusAngular = 0;
    else
        StatusAngular = PrevStatus;
    end
end

%------------------------------------------------------------------------------------------------------------------
%   the different states are as follows:
%   0 = vehicle steady 
%   1 = outside middle circle - integrating deviation of vector
%   2 = inside middle circle on the way back to optimal area 
function StatusLinear = getStatusLinear(Prev_VV_States, VV_States, CircleProps)
    PrevStatus = Prev_VV_States.StatusLinear;
    prevCircle2EEVec = Prev_VV_States.Circle2EEVec;
    VdotP = VV_States.VdotP; 
     Circle2EEVec = VV_States.Circle2EEVec;
    
    if ( PrevStatus == 0 || PrevStatus == 2 ) && norm (Circle2EEVec) > CircleProps.middleCircleRadius && VdotP > 0     
       StatusLinear = 1;
    elseif (PrevStatus == 1 ||  PrevStatus == 2 ) && norm (Circle2EEVec) > CircleProps.middleCircleRadius && VdotP < 0
        StatusLinear = 3;
    elseif (PrevStatus == 1 || PrevStatus == 2) && norm(Circle2EEVec) < CircleProps.middleCircleRadius
        StatusLinear = 3;
    elseif (PrevStatus == 3 || PrevStatus == 2) && norm(Circle2EEVec) < CircleProps.innerCircleRadius
        StatusLinear = 0;
    else
        StatusLinear = PrevStatus;
    end
end

%------------------------------------------------------------------------------------------------------------------
% get the vector to the center of the circle denoted in the
% frame of the center of the circle
function pCircle2EEinFrameC = getPCircle(Kinematics, CircleProps)  
    g0b = Kinematics.Ti.g0b;
    gbe = Kinematics.Ti.gbe;
    circleCenterInFrame0 = g0b(1:3,4) + g0b(1:3,1:3)*CircleProps.CenterInFrameB;
    pVehicle2EEinFrameB = gbe(1:3,4);
    pCircle2EEinFrameC = pVehicle2EEinFrameB - CircleProps.CenterInFrameB;
end

== matlab function Path generator/MATLAB Function1 ==
  data: t input double; gain output double
function gain = fcn(t)
%#codegen
    gain = sin(t*0.5);
    gain = 1;
end

== matlab function Path generator/End Effector2/MATLAB Function1 ==
  data: velocity input double; End_Effector_Com output Bus: endEffector_com_bus; pose input double; pose_quaternion input double
function End_Effector_Com = fcn(velocity,pose, pose_quaternion)
%#codegen
End_Effector_Com = struct('velocity', zeros(6,1), 'pose',zeros(6,1), 'pose_quaternion',zeros(7,1));
End_Effector_Com.pose = pose;
End_Effector_Com.velocity = velocity;
End_Effector_Com.pose_quaternion = pose_quaternion;
end

== matlab function model/End Effector2/MATLAB Function1 ==
  data: velocity input double; End_Effector_Mes output Bus: endEffector_mes_bus; pose input double; pose_quaternion input double
function End_Effector_Mes = fcn(velocity,pose, pose_quaternion)
%#codegen
End_Effector_Mes = struct('velocity', zeros(6,1), 'pose',zeros(6,1), 'pose_quaternion',zeros(7,1));
End_Effector_Mes.pose = pose;
End_Effector_Mes.velocity = velocity;
End_Effector_Mes.pose_quaternion = pose_quaternion;
end

== matlab function Inverse Kinematics/get ee pose error/MATLAB Function1 ==
  data: Kinematics input double; End_Effector_Com input double; e output double; End_Effector_Mes input double
function e = getEE_Error(Kinematics,End_Effector_Com, End_Effector_Mes)
%#codegen
    pose_mes = End_Effector_Mes.pose_quaternion;
    pose_com = End_Effector_Com.pose_quaternion;
    
    Re0 = Kinematics.Ti.R0e';
    
    e = zeros(6,1);
    e(1:3) = pose_com(1:3) - pose_mes(1:3);
    e(4:6) = pose_mes(1)*pose_com(2:4) - pose_com(1)*pose_mes(2:4) - skew(pose_com(2:4))*pose_mes(2:4);
    
    e = [Re0, zeros(3,3) ; zeros(3,3), Re0]*e;
end


function S = skew(v)
  S = [  0   -v(3)  v(2)
       v(3)  0    -v(1)
       -v(2) v(1)   0];
end

== matlab function model/Commanded States/commanded states/Measure States ==
  data: dzeta input double; Commanded_States output Bus: commanded_states_bus; zeta input double; xi input double
function Commanded_States = fcn(dzeta, zeta, xi)
%#codegen

Commanded_States.dzeta = dzeta;
Commanded_States.zeta = zeta;
Commanded_States.xi = xi;

end

== matlab function model/Commanded States/commanded states/zeta2xi/body2eulervel ==
  data: zeta input double size=12; dq output double size=6; dp output double; deuler output double size=3; euler input double
function [dq, dp, deuler] = fcn(zeta, euler)                       
    %#codegen
       
    phi=euler(1);
    theta=euler(2);
    psi=euler(3);
    
    
    cphi = cos(phi);
    sphi = sin(phi);
    cth  = cos(theta);
    sth  = sin(theta);
 
    J1 = Rzyx(phi,theta,psi);
 
    if cth==0, error('J2 is singular for theta = +-90 degrees'); end
 
    J2 = [...
      1  sphi*sth/cth  cphi*sth/cth;
      0  cphi          -sphi;
      0  sphi/cth      cphi/cth ];
 
    J = [ J1  zeros(3,3);
      zeros(3,3) J2 ];
        
    vehicle_velocity_twist = zeta(1:6);

    vehicle_rates=J*vehicle_velocity_twist;
    dp = vehicle_rates(1:3);
    deuler = vehicle_rates(4:6);
    dq = zeta(7:12);
end



function R = Rzyx(phi,theta,psi)
    cphi = cos(phi);
    sphi = sin(phi);
    cth  = cos(theta);
    sth  = sin(theta);
    cpsi = cos(psi);
    spsi = sin(psi);

    R = [...
       cpsi*cth  -spsi*cphi+cpsi*sth*sphi  spsi*sphi+cpsi*cphi*sth
       spsi*cth  cpsi*cphi+sphi*sth*spsi   -cpsi*sphi+sth*spsi*cphi
       -sth      cth*sphi                  cth*cphi ];
end

== matlab function model/End Effector2/twist2pose_quaternions/body2quat ==
  data: ee_velocity_twist input double size=6; ee_rates output double; quat input double
function ee_rates = fcn(ee_velocity_twist, quat)                       
    %#codegen
    
    eta  = quat(1); 
    eps1 = quat(2); 
    eps2 = quat(3); 
    eps3 = quat(4); 
    
    
    normalization_feedback = getNormalizationFeedback(quat);
    
    v = ee_velocity_twist(1:3);
    omega = ee_velocity_twist(4:6);
    
    R = Rquat(quat);

    T = 0.5*[...
    -eps1 -eps2 -eps3        
    eta  -eps3  eps2
    eps3  eta  -eps1
    -eps2  eps1  eta   ];

    pdot = R*v;
    qdot = T*omega + normalization_feedback;
    
    ee_rates = zeros(7,1);
    ee_rates(:) = [pdot; qdot];
    
end



function R = Rquat(q)
%#codegen
eta = q(1);
eps = q(2:4);
S = skew(eps);
R = eye(3) + 2*eta*S + 2*S^2;

end


function S = skew(v)
%#codegen
    S = [  0   -v(3)  v(2)
       v(3)  0    -v(1)
       -v(2) v(1)   0];
end


%----------------------------------------------------------------
%   use normalization feedback according to fossen
%   page 31
%
function q = getNormalizationFeedback(q)
%#codegen
    q = zeros(4,1);
    gamma = 100;
    q = gamma*0.5*(1-q'*q)*q;

end

== matlab function Path generator/End Effector2/twist2pose_euler/body2eulervel ==
  data: ee_velocity_twist input double size=6; ee_rates output double size=6; euler_angles_ee input double size=3
function ee_rates = fcn(ee_velocity_twist, euler_angles_ee)                       
    %#codegen
       
    phi=euler_angles_ee(1);
    theta=euler_angles_ee(2);
    psi=euler_angles_ee(3);
    
    
    cphi = cos(phi);
    sphi = sin(phi);
    cth  = cos(theta);
    sth  = sin(theta);
 
    J1 = Rzyx(phi,theta,psi);
 
    if cth==0, error('J2 is singular for theta = +-90 degrees'); end
 
    J2 = [...
      1  sphi*sth/cth  cphi*sth/cth;
      0  cphi          -sphi;
      0  sphi/cth      cphi/cth ];
 
    J = [ J1  zeros(3,3);
      zeros(3,3) J2 ];
        
    ee_rates = zeros(6,1);
    ee_rates=J*ee_velocity_twist;
end



function R = Rzyx(phi,theta,psi)
    cphi = cos(phi);
    sphi = sin(phi);
    cth  = cos(theta);
    sth  = sin(theta);
    cpsi = cos(psi);
    spsi = sin(psi);

    R = [...
       cpsi*cth  -spsi*cphi+cpsi*sth*sphi  spsi*sphi+cpsi*cphi*sth
       spsi*cth  cpsi*cphi+sphi*sth*spsi   -cpsi*sphi+sth*spsi*cphi
       -sth      cth*sphi                  cth*cphi ];
end

== matlab function Path generator/End Effector2/twist2pose_quaternions/body2quat ==
  data: ee_velocity_twist input double size=6; ee_rates output double; quat input double size=4
function ee_rates = fcn(ee_velocity_twist, quat)                       
    %#codegen
    
    eta  = quat(1); 
    eps1 = quat(2); 
    eps2 = quat(3); 
    eps3 = quat(4); 
    
    
    normalization_feedback = getNormalizationFeedback(quat);
    
    v = ee_velocity_twist(1:3);
    omega = ee_velocity_twist(4:6);
    
    R = Rquat(quat);

    T = 0.5*[...
    -eps1 -eps2 -eps3        
    eta  -eps3  eps2
    eps3  eta  -eps1
    -eps2  eps1  eta   ];

    pdot = R*v;
    qdot = T*omega + normalization_feedback;
    
    ee_rates = zeros(7,1);
    ee_rates(:) = [ pdot ; qdot];
    
    
end



function R = Rquat(q)
%#codegen
eta = q(1);
eps = q(2:4);
S = skew(eps);
R = eye(3) + 2*eta*S + 2*S^2;

end


function S = skew(v)
%#codegen
    S = [  0   -v(3)  v(2)
       v(3)  0    -v(1)
       -v(2) v(1)   0];
end


%----------------------------------------------------------------
%   use normalization feedback according to fossen
%   page 31
%
function q = getNormalizationFeedback(q)
%#codegen
    q = zeros(4,1);
    gamma = 100;
    q = gamma*0.5*(1-q'*q)*q;

end

== matlab function model/End Effector2/twist2pose_quaternions/MATLAB Function ==
  data: pose output double; quaternion output double; poseIn input double
function [pose, quaternion] = fcn(poseIn)
%#codegen
    pose = poseIn;
    quaternion = poseIn(4:7);
end

== matlab function Path generator/End Effector2/twist2pose_quaternions/MATLAB Function ==
  data: pose output double; quaternion output double; poseIn input double
function [pose, quaternion] = fcn(poseIn)
%#codegen
    pose = poseIn;
    quaternion = poseIn(4:7);
end

== matlab function Inverse Kinematics/get ee pose error/MATLAB Function2 ==
  data: End_Effector_Com input double; e output double; End_Effector_Mes input double
function e = getEEVelError(End_Effector_Com, End_Effector_Mes)
    e = End_Effector_Com.velocity - End_Effector_Mes.velocity;
end

== matlab function Path generator/MATLAB Function2 ==
  data: Kinematics input double; V input double; Vout output double
function Vout = fcn(Kinematics, V)
%#codegen
Adg0e_inv = Kinematics.Ti.Adg0e_inv ;
Re0 = Kinematics.Ti.R0e';
Vout = [Re0, zeros(3,3) ; zeros(3,3) , Re0] * V;

end
